simulink model "sys2order"  (Simulink 8.1)
settings: Solver=ode23  StartTime=0.0  StopTime=15  FixedStep=dt  RelTol=1e-3
values from neighbouring files (symbols this model uses):
  A = [-2 1;-1 0]    [RT_dennis_draussen.m]    (also in RT_klausurvorb.m = [0 0; 1 -3]; RT_ueb2_proc.m = [0 1; -2 -3]; sys2order_post.m = [0 1;0 -(R*rho+psi)/(R*J)])
  b = [-2;1]    [RT_dennis_draussen.m]    (also in RT_klausurvorb.m = [1;0]; RT_sys_2nd_order_post.m = 5; RT_ueb2_proc.m = [0;3]; sys2order_post.m = [0;1/(J*R)])
  c = [0 3*.65]    [RT_klausurvorb.m]    (also in RT_ueb2_proc.m = [1;0]'; sys2order_post.m = [1,0])
  d = 1    [RT_dennis_draussen.m]    (also in RT_klausurvorb.m = 0; RT_reglersynthesePDF.m = strsplit(int2str(GsKp.den{1})); RT_ueb2_proc.m = 0; regelungstechnik.m = 0.08)
  x0 = [1;2]    [RT_ueb2_proc.m]    (also in sys2order_post.m = [0;0])
settings Model: Creator=mainster  LastModifiedBy=mainster

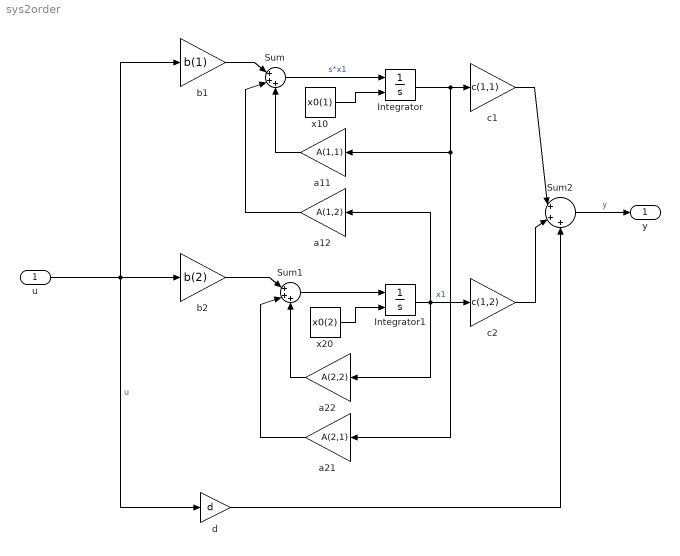
== system sys2order ==
  u : Inport
  Integrator : Integrator  InitialConditionSource=external
  Integrator1 : Integrator  InitialConditionSource=external
  Sum : Sum  Inputs=|+++
  Sum1 : Sum  Inputs=|+++
  Sum2 : Sum  Inputs=|+++
  a11 : Gain  Gain=A(1,1)  RndMeth=Round
  a12 : Gain  Gain=A(1,2)  RndMeth=Round
  a21 : Gain  Gain=A(2,1)  RndMeth=Round
  a22 : Gain  Gain=A(2,2)  RndMeth=Round
  b1 : Gain  Gain=b(1)  RndMeth=Round
  b2 : Gain  Gain=b(2)  RndMeth=Round
  c1 : Gain  Gain=c(1,1)  RndMeth=Round
  c2 : Gain  Gain=c(1,2)  RndMeth=Round
  d : Gain  Gain=d
  x10 : Constant  Value=x0(1)
  x20 : Constant  Value=x0(2)
  y : Outport
  wires:
  b2/1 -> Sum1/1
  a21/1 -> Sum1/2
  a22/1 -> Sum1/3
  b1/1 -> Sum/1
  a12/1 -> Sum/2
  a11/1 -> Sum/3
  Sum/1 -> Integrator/1  "s*x1"
  Sum1/1 -> Integrator1/1
  x20/1 -> Integrator1/2
  x10/1 -> Integrator/2
  Integrator1/1 -> a22/1, c2/1, a12/1
  Integrator/1 -> a11/1, a21/1, c1/1  "x1"
  c1/1 -> Sum2/1
  c2/1 -> Sum2/2
  u/1 -> b1/1, d/1, b2/1  "u"
  d/1 -> Sum2/3
  Sum2/1 -> y/1  "y"
